simulink model "truth_plant"  (R2025b)
settings: Solver=FixedStepAuto  StartTime=0.0  StopTime=70.0  FixedStep=0.05  RelTol=1e-3
settings Model: Creator=Ricardo  LastModifiedBy=Ricardo

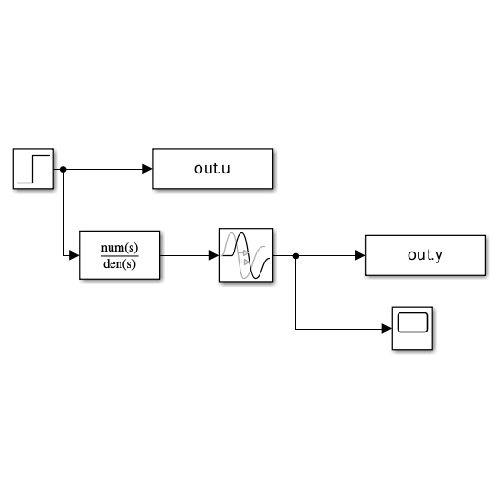
[thumbnail: Simulink's stored preview of the top-level diagram]
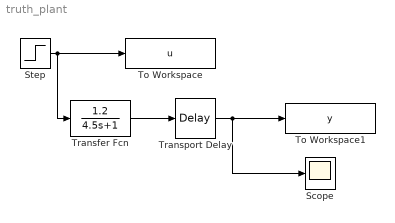
== system truth_plant ==
  Scope : Scope
      settings: ActiveDisplayYMinimum=-0.15331286847526174  ActiveDisplayYMaximum=0.71490423702687622
  Step : Step  Time=10  After=0.5  SampleTime=0
  To Workspace : ToWorkspace  VariableName=u  SampleTime=-1
  To Workspace1 : ToWorkspace  VariableName=y  SampleTime=-1
  Transfer Fcn : TransferFcn  Numerator=[1.2]  Denominator=[4.5 1]
  Transport Delay : TransportDelay  DelayTime=0.8
  wires:
  Step/1 -> Transfer Fcn/1, To Workspace/1
  Transfer Fcn/1 -> Transport Delay/1
  Transport Delay/1 -> Scope/1, To Workspace1/1
